simulink model "P2Q1"  (R2018a)
settings: Solver=VariableStepAuto  StartTime=0.0  StopTime=10.0  RelTol=1e-3
libraries: dspstat3 x3, dspmathops x3, dsparch4 x2, dspsrcs4 x1, simulink x1
settings Model: Creator=Marine  LastModifiedBy=ifaruk

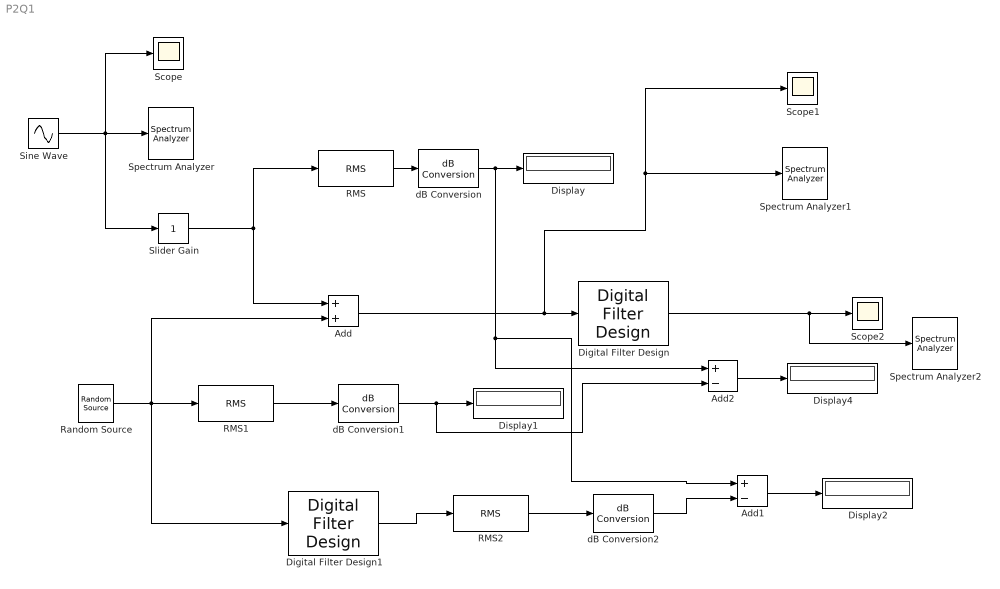
== system P2Q1 ==
  Add : Sum
  Add1 : Sum  Inputs=+-
  Add2 : Sum  Inputs=+-
  Digital Filter Design : dsparch4/Digital Filter Design  mwdsp_browser_bugfix_var=off
  Digital Filter Design1 : dsparch4/Digital Filter Design  mwdsp_browser_bugfix_var=off
  Display{,1..2,4} (4 alike) : Display
  RMS : dspstat3/RMS  run=on  directionMode=Each column  dimension=1  reset_popup=None
  RMS1 : dspstat3/RMS  run=on  directionMode=Each column  dimension=1  reset_popup=None
  RMS2 : dspstat3/RMS  run=on  directionMode=Each column  dimension=1  reset_popup=None
  Random Source : dspsrcs4/Random Source  SrcType=Gaussian  NormMethod=Ziggurat  CltLength=12  MinVal=0  MaxVal=1  MeanVal=0  VarVal=1  RepMode=Not repeatable  rawSeed=1  IsInherit=off  SampMode=Discrete  SampTime=0.0001  SampFrame=1  DataType=Double  OutComplex=Real  OutputFrames=off
  Scope : Scope
  Scope1 : Scope
  Scope2 : Scope
  Sine Wave : Sin  SineType=Sample based  Samples=100  SampleTime=0.0001
  Slider Gain : simulink/Math Operations/Slider Gain  gain=1  low=0  high=2
  Spectrum Analyzer : SpectrumAnalyzer
  Spectrum Analyzer1 : SpectrumAnalyzer
  Spectrum Analyzer2 : SpectrumAnalyzer
  dB Conversion : dspmathops/dB Conversion  dBtype=dB  intype=Amplitude  R=1  fuzz=off
      settings: SourceProductName=DSP System Toolbox
  dB Conversion1 : dspmathops/dB Conversion  dBtype=dB  intype=Amplitude  R=1  fuzz=off
      settings: SourceProductName=DSP System Toolbox
  dB Conversion2 : dspmathops/dB Conversion  dBtype=dB  intype=Amplitude  R=1  fuzz=off
      settings: SourceProductName=DSP System Toolbox
  wires:
  Sine Wave/1 -> Slider Gain/1, Spectrum Analyzer/1, Scope/1
  Slider Gain/1 -> Add/1, RMS/1
  RMS/1 -> dB Conversion/1
  dB Conversion/1 -> Add1/1, Add2/1, Display/1
  Random Source/1 -> Add/2, Digital Filter Design1/1, RMS1/1
  RMS1/1 -> dB Conversion1/1
  dB Conversion1/1 -> Add2/2, Display1/1
  Digital Filter Design1/1 -> RMS2/1
  RMS2/1 -> dB Conversion2/1
  Add1/1 -> Display2/1
  dB Conversion2/1 -> Add1/2
  Add/1 -> Scope1/1, Spectrum Analyzer1/1, Digital Filter Design/1
  Digital Filter Design/1 -> Spectrum Analyzer2/1, Scope2/1
  Add2/1 -> Display4/1
